simulink model "sim_sys2"  (R2013b)
settings: Solver=ode45  StartTime=0.0  StopTime=5000  RelTol=1e-3
undefined symbols (not defined in the file or in its folder): msdft_comb, resonator, sys_lib, twiddle_factors
libraries: xbsIndex_r4 x3996, casper_library_misc x310, xps_library x1
(part 1 of 46)
settings Model: Creator=root  LastModifiedBy=root

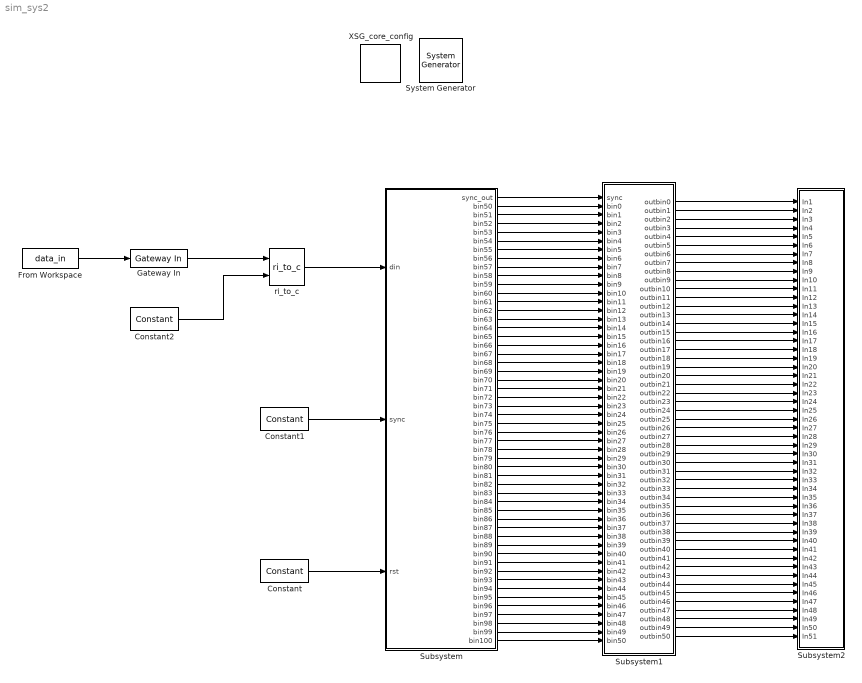
== system sim_sys2 ==
  " System Generator" : xbsIndex_r4/ System Generator  Tag=genX  xilinxfamily=Kintex7  part=xc7k325t  speed=-3  package=fbg676  synthesis_tool=XST  clock_wrapper=Clock Enables  directory=./netlist  proj_type=Project Navigator  Synth_file=XST Defaults  Impl_file=ISE Defaults  testbench=off  simulink_period=1  sysclk_period=10  dcm_input_clock_period=10  incr_netlist=off  trim_vbits=Everywhere in SubSystem  dbl_ovrd=According to Block Masks  core_generation=According to Block Masks  run_coregen=off  deprecated_control=off  eval_field=0  block_type=sysgen
  Constant : xbsIndex_r4/Constant  const=0  gui_display_data_type=Boolean  arith_type=Boolean  n_bits=16  bin_pt=14  preci_type=Single  exp_width=8  frac_width=24  explicit_period=on  period=1  equ=P=C  opselect=C  inp2=PCIN>>17  opr=+  inp1=P  carry=CIN  dbl_ovrd=off  block_type=constant
  Constant1 : xbsIndex_r4/Constant  const=1  gui_display_data_type=Boolean  arith_type=Boolean  n_bits=16  bin_pt=14  preci_type=Single  exp_width=8  frac_width=24  explicit_period=on  period=1  equ=P=C  opselect=C  inp2=PCIN>>17  opr=+  inp1=P  carry=CIN  dbl_ovrd=off  block_type=constant
  Constant2 : xbsIndex_r4/Constant  const=0  gui_display_data_type=Fixed-point  arith_type=Signed (2's comp)  n_bits=10  bin_pt=9  preci_type=Single  exp_width=8  frac_width=24  explicit_period=on  period=1  equ=P=C  opselect=C  inp2=PCIN>>17  opr=+  inp1=P  carry=CIN  dbl_ovrd=off  block_type=constant
  From Workspace : FromWorkspace  VariableName=data_in  SampleTime=0
  Gateway In : xbsIndex_r4/Gateway In  gui_display_data_type=Fixed-point  arith_type="Signed  (2's comp)"  n_bits=10  bin_pt=9  preci_type=Single  exp_width=8  frac_width=24  quantization="Round  (unbiased: +/- Inf)"  overflow=Saturate  period=1  dbl_ovrd=off  timing_constraint=None  locs_specified=off  LOCs={}  UseAsADC=off  ADCChannel='1'  inherit_from_input=off  hdl_port=on  block_type=gatewayin
  Subsystem : Subsystem  mask{input_bitsize=10, fft_len=10, bin_range=[50:1:100], twid_bitsize=15, res_out_size=40, out_bitsize=60, latency=0}
      mask prompts: input_bitsize "input bitsize"; fft_len "fft len (2^?)"; bin_range "bins"; res_out_size "resonator output"
      mask init:
      | config.source = str2func('msdft2_init');
      | config.toplevel = gcb;
      | xBlock(config, {input_bitsize, fft_len, bin_range,...
      |             twid_bitsize, res_out_size, ...
      |             out_bitsize, latency});
  Subsystem1 : Subsystem  mask{bin_len=51, bitwidth=40}
      mask prompts: bin_len "bin length"; bitwidth "bit width"
      mask init:
      | config.source = str2func('init_gate');
      | config.toplevel = gcb;
      | xBlock(config, {bin_len, bitwidth});
  Subsystem2 : Subsystem
  XSG_core_config : xps_library/XSG_core_config  Tag=xps:xsg  hw_sys=ROACH2:sx475t  clk_src=sys_clk  ROACH_clk_src=sys_clk  ROACH2_clk_src=sys_clk  MKDIG_clk_src=sys_clk  clk_rate=100  sample_period=1  synthesis_tool=XST
  ri_to_c : casper_library_misc/ri_to_c
  wires:
  Subsystem/52(bin100) -> Subsystem1/52(bin50)
  Subsystem/51(bin99) -> Subsystem1/51(bin49)
  Subsystem/50(bin98) -> Subsystem1/50(bin48)
  Subsystem/49(bin97) -> Subsystem1/49(bin47)
  Subsystem/48(bin96) -> Subsystem1/48(bin46)
  Subsystem/47(bin95) -> Subsystem1/47(bin45)
  Subsystem/45(bin93) -> Subsystem1/45(bin43)
  Subsystem/46(bin94) -> Subsystem1/46(bin44)
  Subsystem/44(bin92) -> Subsystem1/44(bin42)
  Subsystem/43(bin91) -> Subsystem1/43(bin41)
  Subsystem/42(bin90) -> Subsystem1/42(bin40)
  Subsystem/41(bin89) -> Subsystem1/41(bin39)
  Subsystem/40(bin88) -> Subsystem1/40(bin38)
  Subsystem/39(bin87) -> Subsystem1/39(bin37)
  Subsystem/38(bin86) -> Subsystem1/38(bin36)
  Subsystem/37(bin85) -> Subsystem1/37(bin35)
  Subsystem/36(bin84) -> Subsystem1/36(bin34)
  Subsystem/35(bin83) -> Subsystem1/35(bin33)
  Subsystem/34(bin82) -> Subsystem1/34(bin32)
  Subsystem/33(bin81) -> Subsystem1/33(bin31)
  Subsystem/32(bin80) -> Subsystem1/32(bin30)
  Subsystem/31(bin79) -> Subsystem1/31(bin29)
  Subsystem/30(bin78) -> Subsystem1/30(bin28)
  Subsystem/29(bin77) -> Subsystem1/29(bin27)
  Subsystem/28(bin76) -> Subsystem1/28(bin26)
  Subsystem/27(bin75) -> Subsystem1/27(bin25)
  Subsystem/26(bin74) -> Subsystem1/26(bin24)
  Subsystem/25(bin73) -> Subsystem1/25(bin23)
  Subsystem/24(bin72) -> Subsystem1/24(bin22)
  Subsystem/23(bin71) -> Subsystem1/23(bin21)
  Subsystem/22(bin70) -> Subsystem1/22(bin20)
  Subsystem/21(bin69) -> Subsystem1/21(bin19)
  Subsystem/20(bin68) -> Subsystem1/20(bin18)
  Subsystem/19(bin67) -> Subsystem1/19(bin17)
  Subsystem/18(bin66) -> Subsystem1/18(bin16)
  Subsystem/17(bin65) -> Subsystem1/17(bin15)
  Subsystem/16(bin64) -> Subsystem1/16(bin14)
  Subsystem/15(bin63) -> Subsystem1/15(bin13)
  Subsystem/14(bin62) -> Subsystem1/14(bin12)
  Subsystem/13(bin61) -> Subsystem1/13(bin11)
  Subsystem/12(bin60) -> Subsystem1/12(bin10)
  Subsystem/11(bin59) -> Subsystem1/11(bin9)
  Subsystem/10(bin58) -> Subsystem1/10(bin8)
  Subsystem/9(bin57) -> Subsystem1/9(bin7)
  Subsystem/8(bin56) -> Subsystem1/8(bin6)
  Subsystem/7(bin55) -> Subsystem1/7(bin5)
  Subsystem/6(bin54) -> Subsystem1/6(bin4)
  Subsystem/5(bin53) -> Subsystem1/5(bin3)
  Subsystem/4(bin52) -> Subsystem1/4(bin2)
  Subsystem/3(bin51) -> Subsystem1/3(bin1)
  Subsystem/2(bin50) -> Subsystem1/2(bin0)
  Subsystem/1(sync_out) -> Subsystem1/1(sync)
  Constant/1 -> Subsystem/3(rst)
  Constant1/1 -> Subsystem/2(sync)
  ri_to_c/1 -> Subsystem/1(din)
  Gateway In/1 -> ri_to_c/1
  From Workspace/1 -> Gateway In/1
  Constant2/1 -> ri_to_c/2
  Subsystem1/26(outbin25) -> Subsystem2/26(In26)
  Subsystem1/19(outbin18) -> Subsystem2/19(In19)
  Subsystem1/20(outbin19) -> Subsystem2/20(In20)
  Subsystem1/37(outbin36) -> Subsystem2/37(In37)
  Subsystem1/49(outbin48) -> Subsystem2/49(In49)
  Subsystem1/45(outbin44) -> Subsystem2/45(In45)
  Subsystem1/32(outbin31) -> Subsystem2/32(In32)
  Subsystem1/6(outbin5) -> Subsystem2/6(In6)
  Subsystem1/44(outbin43) -> Subsystem2/44(In44)
  Subsystem1/39(outbin38) -> Subsystem2/39(In39)
  Subsystem1/15(outbin14) -> Subsystem2/15(In15)
  Subsystem1/14(outbin13) -> Subsystem2/14(In14)
  Subsystem1/11(outbin10) -> Subsystem2/11(In11)
  Subsystem1/50(outbin49) -> Subsystem2/50(In50)
  Subsystem1/2(outbin1) -> Subsystem2/2(In2)
  Subsystem1/38(outbin37) -> Subsystem2/38(In38)
  Subsystem1/23(outbin22) -> Subsystem2/23(In23)
  Subsystem1/51(outbin50) -> Subsystem2/51(In51)
  Subsystem1/3(outbin2) -> Subsystem2/3(In3)
  Subsystem1/41(outbin40) -> Subsystem2/41(In41)
  Subsystem1/40(outbin39) -> Subsystem2/40(In40)
  Subsystem1/4(outbin3) -> Subsystem2/4(In4)
  Subsystem1/36(outbin35) -> Subsystem2/36(In36)
  Subsystem1/1(outbin0) -> Subsystem2/1(In1)
  Subsystem1/9(outbin8) -> Subsystem2/9(In9)
  Subsystem1/31(outbin30) -> Subsystem2/31(In31)
  Subsystem1/17(outbin16) -> Subsystem2/17(In17)
  Subsystem1/46(outbin45) -> Subsystem2/46(In46)
  Subsystem1/35(outbin34) -> Subsystem2/35(In35)
  Subsystem1/5(outbin4) -> Subsystem2/5(In5)
  Subsystem1/22(outbin21) -> Subsystem2/22(In22)
  Subsystem1/12(outbin11) -> Subsystem2/12(In12)
  Subsystem1/33(outbin32) -> Subsystem2/33(In33)
  Subsystem1/13(outbin12) -> Subsystem2/13(In13)
  Subsystem1/24(outbin23) -> Subsystem2/24(In24)
  Subsystem1/34(outbin33) -> Subsystem2/34(In34)
  Subsystem1/47(outbin46) -> Subsystem2/47(In47)
  Subsystem1/27(outbin26) -> Subsystem2/27(In27)
  Subsystem1/30(outbin29) -> Subsystem2/30(In30)
  Subsystem1/43(outbin42) -> Subsystem2/43(In43)
  Subsystem1/10(outbin9) -> Subsystem2/10(In10)
  Subsystem1/28(outbin27) -> Subsystem2/28(In28)
  Subsystem1/42(outbin41) -> Subsystem2/42(In42)
  Subsystem1/21(outbin20) -> Subsystem2/21(In21)
  Subsystem1/16(outbin15) -> Subsystem2/16(In16)
  Subsystem1/25(outbin24) -> Subsystem2/25(In25)
  Subsystem1/18(outbin17) -> Subsystem2/18(In18)
  Subsystem1/29(outbin28) -> Subsystem2/29(In29)
  Subsystem1/8(outbin7) -> Subsystem2/8(In8)
  Subsystem1/7(outbin6) -> Subsystem2/7(In7)
  Subsystem1/48(outbin47) -> Subsystem2/48(In48)

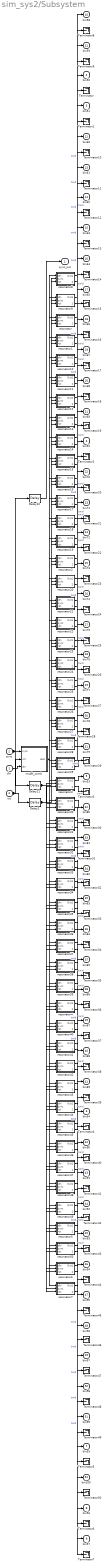
== system sim_sys2/Subsystem ==
  din : Inport
  sync : Inport  Port=2
  rst : Inport  Port=3
  Delay2 : xbsIndex_r4/Delay  rst=off  infoeditControl=Selection of Reset will increase slice count due to use of real FFs and instead of SRLs  en=off  latency=1  dbl_ovrd=off  reg_retiming=off  block_type=delay
  Delay21 : xbsIndex_r4/Delay  rst=off  infoeditControl=Selection of Reset will increase slice count due to use of real FFs and instead of SRLs  en=off  latency=1  dbl_ovrd=off  reg_retiming=off  block_type=delay
  Delay22 : xbsIndex_r4/Delay  rst=off  infoeditControl=Selection of Reset will increase slice count due to use of real FFs and instead of SRLs  en=off  latency=1036  dbl_ovrd=off  reg_retiming=off  block_type=delay
  Terminator{,1..50} (51 alike) : Terminator
  msdft_comb : Subsystem  AncestorBlock=sys_lib/msdft_comb  mask(msdft_comb){input_bitsize=10, fft_len=10, latency=0}
      mask prompts: fft_len "fft_len (2^?)"; latency "sub latency"
      mask init:
      | msdft_comb_init(gcb, ...
      |         'input_bitsize', input_bitsize, ...
      |         'fft_len', fft_len, ...
      |         'latency', latency);
      settings: AttributesFormatString=latency=0
  resonator : Subsystem  AncestorBlock=sys_lib/resonator  mask(msdft_res){fft_len=10, twid_bitsize=15, bin_number=50, input_bitsize=11, input_frac=9, res_bitsize=40, add_lat=0}
      mask prompts: fft_len "fft len(2^?)"; twid_bitsize "twid bitsize"; bin_number "bin number"; input_bitsize "input bitsize"; input_frac "input frac"; res_bitsize "out resonator size"
      mask init:
      | msdft_resonator_init(gcb, ...
      |                 'fft_len', fft_len, ...
      |                 'twid_bitsize', twid_bitsize, ...
      |                 'bin_number', bin_number, ...
      |                 'input_bitsize', input_bitsize, ...
      |                 'input_frac', input_frac, ...
      |                 'res_bitsize', res_bitsize, ...
      |                 'add_lat', add_lat);
      settings: AttributesFormatString=N=10, k=50
  resonator1 : Subsystem  AncestorBlock=sys_lib/resonator  mask(msdft_res){fft_len=10, twid_bitsize=15, bin_number=51, input_bitsize=11, input_frac=9, res_bitsize=40, add_lat=0}
      mask prompts: fft_len "fft len(2^?)"; twid_bitsize "twid bitsize"; bin_number "bin number"; input_bitsize "input bitsize"; input_frac "input frac"; res_bitsize "out resonator size"
      mask init: same as sim_sys2/Subsystem/resonator
      settings: AttributesFormatString=N=10, k=51
  resonator10 : Subsystem  AncestorBlock=sys_lib/resonator  mask(msdft_res){fft_len=10, twid_bitsize=15, bin_number=60, input_bitsize=11, input_frac=9, res_bitsize=40, add_lat=0}
      mask prompts: fft_len "fft len(2^?)"; twid_bitsize "twid bitsize"; bin_number "bin number"; input_bitsize "input bitsize"; input_frac "input frac"; res_bitsize "out resonator size"
      mask init: same as sim_sys2/Subsystem/resonator
      settings: AttributesFormatString=N=10, k=60
  resonator11 : Subsystem  AncestorBlock=sys_lib/resonator  mask(msdft_res){fft_len=10, twid_bitsize=15, bin_number=61, input_bitsize=11, input_frac=9, res_bitsize=40, add_lat=0}
      mask prompts: fft_len "fft len(2^?)"; twid_bitsize "twid bitsize"; bin_number "bin number"; input_bitsize "input bitsize"; input_frac "input frac"; res_bitsize "out resonator size"
      mask init: same as sim_sys2/Subsystem/resonator
      settings: AttributesFormatString=N=10, k=61
  resonator12 : Subsystem  AncestorBlock=sys_lib/resonator  mask(msdft_res){fft_len=10, twid_bitsize=15, bin_number=62, input_bitsize=11, input_frac=9, res_bitsize=40, add_lat=0}
      mask prompts: fft_len "fft len(2^?)"; twid_bitsize "twid bitsize"; bin_number "bin number"; input_bitsize "input bitsize"; input_frac "input frac"; res_bitsize "out resonator size"
      mask init: same as sim_sys2/Subsystem/resonator
      settings: AttributesFormatString=N=10, k=62
  resonator13 : Subsystem  AncestorBlock=sys_lib/resonator  mask(msdft_res){fft_len=10, twid_bitsize=15, bin_number=63, input_bitsize=11, input_frac=9, res_bitsize=40, add_lat=0}
      mask prompts: fft_len "fft len(2^?)"; twid_bitsize "twid bitsize"; bin_number "bin number"; input_bitsize "input bitsize"; input_frac "input frac"; res_bitsize "out resonator size"
      mask init: same as sim_sys2/Subsystem/resonator
      settings: AttributesFormatString=N=10, k=63
  resonator14 : Subsystem  AncestorBlock=sys_lib/resonator  mask(msdft_res){fft_len=10, twid_bitsize=15, bin_number=64, input_bitsize=11, input_frac=9, res_bitsize=40, add_lat=0}
      mask prompts: fft_len "fft len(2^?)"; twid_bitsize "twid bitsize"; bin_number "bin number"; input_bitsize "input bitsize"; input_frac "input frac"; res_bitsize "out resonator size"
      mask init: same as sim_sys2/Subsystem/resonator
      settings: AttributesFormatString=N=10, k=64
  resonator15 : Subsystem  AncestorBlock=sys_lib/resonator  mask(msdft_res){fft_len=10, twid_bitsize=15, bin_number=65, input_bitsize=11, input_frac=9, res_bitsize=40, add_lat=0}
      mask prompts: fft_len "fft len(2^?)"; twid_bitsize "twid bitsize"; bin_number "bin number"; input_bitsize "input bitsize"; input_frac "input frac"; res_bitsize "out resonator size"
      mask init: same as sim_sys2/Subsystem/resonator
      settings: AttributesFormatString=N=10, k=65
  resonator16 : Subsystem  AncestorBlock=sys_lib/resonator  mask(msdft_res){fft_len=10, twid_bitsize=15, bin_number=66, input_bitsize=11, input_frac=9, res_bitsize=40, add_lat=0}
      mask prompts: fft_len "fft len(2^?)"; twid_bitsize "twid bitsize"; bin_number "bin number"; input_bitsize "input bitsize"; input_frac "input frac"; res_bitsize "out resonator size"
      mask init: same as sim_sys2/Subsystem/resonator
      settings: AttributesFormatString=N=10, k=66
  resonator17 : Subsystem  AncestorBlock=sys_lib/resonator  mask(msdft_res){fft_len=10, twid_bitsize=15, bin_number=67, input_bitsize=11, input_frac=9, res_bitsize=40, add_lat=0}
      mask prompts: fft_len "fft len(2^?)"; twid_bitsize "twid bitsize"; bin_number "bin number"; input_bitsize "input bitsize"; input_frac "input frac"; res_bitsize "out resonator size"
      mask init: same as sim_sys2/Subsystem/resonator
      settings: AttributesFormatString=N=10, k=67
  resonator18 : Subsystem  AncestorBlock=sys_lib/resonator  mask(msdft_res){fft_len=10, twid_bitsize=15, bin_number=68, input_bitsize=11, input_frac=9, res_bitsize=40, add_lat=0}
      mask prompts: fft_len "fft len(2^?)"; twid_bitsize "twid bitsize"; bin_number "bin number"; input_bitsize "input bitsize"; input_frac "input frac"; res_bitsize "out resonator size"
      mask init: same as sim_sys2/Subsystem/resonator
      settings: AttributesFormatString=N=10, k=68
  resonator19 : Subsystem  AncestorBlock=sys_lib/resonator  mask(msdft_res){fft_len=10, twid_bitsize=15, bin_number=69, input_bitsize=11, input_frac=9, res_bitsize=40, add_lat=0}
      mask prompts: fft_len "fft len(2^?)"; twid_bitsize "twid bitsize"; bin_number "bin number"; input_bitsize "input bitsize"; input_frac "input frac"; res_bitsize "out resonator size"
      mask init: same as sim_sys2/Subsystem/resonator
      settings: AttributesFormatString=N=10, k=69
  resonator2 : Subsystem  AncestorBlock=sys_lib/resonator  mask(msdft_res){fft_len=10, twid_bitsize=15, bin_number=52, input_bitsize=11, input_frac=9, res_bitsize=40, add_lat=0}
      mask prompts: fft_len "fft len(2^?)"; twid_bitsize "twid bitsize"; bin_number "bin number"; input_bitsize "input bitsize"; input_frac "input frac"; res_bitsize "out resonator size"
      mask init: same as sim_sys2/Subsystem/resonator
      settings: AttributesFormatString=N=10, k=52
  resonator20 : Subsystem  AncestorBlock=sys_lib/resonator  mask(msdft_res){fft_len=10, twid_bitsize=15, bin_number=70, input_bitsize=11, input_frac=9, res_bitsize=40, add_lat=0}
      mask prompts: fft_len "fft len(2^?)"; twid_bitsize "twid bitsize"; bin_number "bin number"; input_bitsize "input bitsize"; input_frac "input frac"; res_bitsize "out resonator size"
      mask init: same as sim_sys2/Subsystem/resonator
      settings: AttributesFormatString=N=10, k=70
  resonator21 : Subsystem  AncestorBlock=sys_lib/resonator  mask(msdft_res){fft_len=10, twid_bitsize=15, bin_number=71, input_bitsize=11, input_frac=9, res_bitsize=40, add_lat=0}
      mask prompts: fft_len "fft len(2^?)"; twid_bitsize "twid bitsize"; bin_number "bin number"; input_bitsize "input bitsize"; input_frac "input frac"; res_bitsize "out resonator size"
      mask init: same as sim_sys2/Subsystem/resonator
      settings: AttributesFormatString=N=10, k=71
  resonator22 : Subsystem  AncestorBlock=sys_lib/resonator  mask(msdft_res){fft_len=10, twid_bitsize=15, bin_number=72, input_bitsize=11, input_frac=9, res_bitsize=40, add_lat=0}
      mask prompts: fft_len "fft len(2^?)"; twid_bitsize "twid bitsize"; bin_number "bin number"; input_bitsize "input bitsize"; input_frac "input frac"; res_bitsize "out resonator size"
      mask init: same as sim_sys2/Subsystem/resonator
      settings: AttributesFormatString=N=10, k=72
  resonator23 : Subsystem  AncestorBlock=sys_lib/resonator  mask(msdft_res){fft_len=10, twid_bitsize=15, bin_number=73, input_bitsize=11, input_frac=9, res_bitsize=40, add_lat=0}
      mask prompts: fft_len "fft len(2^?)"; twid_bitsize "twid bitsize"; bin_number "bin number"; input_bitsize "input bitsize"; input_frac "input frac"; res_bitsize "out resonator size"
      mask init: same as sim_sys2/Subsystem/resonator
      settings: AttributesFormatString=N=10, k=73
  resonator24 : Subsystem  AncestorBlock=sys_lib/resonator  mask(msdft_res){fft_len=10, twid_bitsize=15, bin_number=74, input_bitsize=11, input_frac=9, res_bitsize=40, add_lat=0}
      mask prompts: fft_len "fft len(2^?)"; twid_bitsize "twid bitsize"; bin_number "bin number"; input_bitsize "input bitsize"; input_frac "input frac"; res_bitsize "out resonator size"
      mask init: same as sim_sys2/Subsystem/resonator
      settings: AttributesFormatString=N=10, k=74
  resonator25 : Subsystem  AncestorBlock=sys_lib/resonator  mask(msdft_res){fft_len=10, twid_bitsize=15, bin_number=75, input_bitsize=11, input_frac=9, res_bitsize=40, add_lat=0}
      mask prompts: fft_len "fft len(2^?)"; twid_bitsize "twid bitsize"; bin_number "bin number"; input_bitsize "input bitsize"; input_frac "input frac"; res_bitsize "out resonator size"
      mask init: same as sim_sys2/Subsystem/resonator
      settings: AttributesFormatString=N=10, k=75
  resonator26 : Subsystem  AncestorBlock=sys_lib/resonator  mask(msdft_res){fft_len=10, twid_bitsize=15, bin_number=76, input_bitsize=11, input_frac=9, res_bitsize=40, add_lat=0}
      mask prompts: fft_len "fft len(2^?)"; twid_bitsize "twid bitsize"; bin_number "bin number"; input_bitsize "input bitsize"; input_frac "input frac"; res_bitsize "out resonator size"
      mask init: same as sim_sys2/Subsystem/resonator
      settings: AttributesFormatString=N=10, k=76
  resonator27 : Subsystem  AncestorBlock=sys_lib/resonator  mask(msdft_res){fft_len=10, twid_bitsize=15, bin_number=77, input_bitsize=11, input_frac=9, res_bitsize=40, add_lat=0}
      mask prompts: fft_len "fft len(2^?)"; twid_bitsize "twid bitsize"; bin_number "bin number"; input_bitsize "input bitsize"; input_frac "input frac"; res_bitsize "out resonator size"
      mask init: same as sim_sys2/Subsystem/resonator
      settings: AttributesFormatString=N=10, k=77
  resonator28 : Subsystem  AncestorBlock=sys_lib/resonator  mask(msdft_res){fft_len=10, twid_bitsize=15, bin_number=78, input_bitsize=11, input_frac=9, res_bitsize=40, add_lat=0}
      mask prompts: fft_len "fft len(2^?)"; twid_bitsize "twid bitsize"; bin_number "bin number"; input_bitsize "input bitsize"; input_frac "input frac"; res_bitsize "out resonator size"
      mask init: same as sim_sys2/Subsystem/resonator
      settings: AttributesFormatString=N=10, k=78
  resonator29 : Subsystem  AncestorBlock=sys_lib/resonator  mask(msdft_res){fft_len=10, twid_bitsize=15, bin_number=79, input_bitsize=11, input_frac=9, res_bitsize=40, add_lat=0}
      mask prompts: fft_len "fft len(2^?)"; twid_bitsize "twid bitsize"; bin_number "bin number"; input_bitsize "input bitsize"; input_frac "input frac"; res_bitsize "out resonator size"
      mask init: same as sim_sys2/Subsystem/resonator
      settings: AttributesFormatString=N=10, k=79
  resonator3 : Subsystem  AncestorBlock=sys_lib/resonator  mask(msdft_res){fft_len=10, twid_bitsize=15, bin_number=53, input_bitsize=11, input_frac=9, res_bitsize=40, add_lat=0}
      mask prompts: fft_len "fft len(2^?)"; twid_bitsize "twid bitsize"; bin_number "bin number"; input_bitsize "input bitsize"; input_frac "input frac"; res_bitsize "out resonator size"
      mask init: same as sim_sys2/Subsystem/resonator
      settings: AttributesFormatString=N=10, k=53
  resonator30 : Subsystem  AncestorBlock=sys_lib/resonator  mask(msdft_res){fft_len=10, twid_bitsize=15, bin_number=80, input_bitsize=11, input_frac=9, res_bitsize=40, add_lat=0}
      mask prompts: fft_len "fft len(2^?)"; twid_bitsize "twid bitsize"; bin_number "bin number"; input_bitsize "input bitsize"; input_frac "input frac"; res_bitsize "out resonator size"
      mask init: same as sim_sys2/Subsystem/resonator
      settings: AttributesFormatString=N=10, k=80
  resonator31 : Subsystem  AncestorBlock=sys_lib/resonator  mask(msdft_res){fft_len=10, twid_bitsize=15, bin_number=81, input_bitsize=11, input_frac=9, res_bitsize=40, add_lat=0}
      mask prompts: fft_len "fft len(2^?)"; twid_bitsize "twid bitsize"; bin_number "bin number"; input_bitsize "input bitsize"; input_frac "input frac"; res_bitsize "out resonator size"
      mask init: same as sim_sys2/Subsystem/resonator
      settings: AttributesFormatString=N=10, k=81
  resonator32 : Subsystem  AncestorBlock=sys_lib/resonator  mask(msdft_res){fft_len=10, twid_bitsize=15, bin_number=82, input_bitsize=11, input_frac=9, res_bitsize=40, add_lat=0}
      mask prompts: fft_len "fft len(2^?)"; twid_bitsize "twid bitsize"; bin_number "bin number"; input_bitsize "input bitsize"; input_frac "input frac"; res_bitsize "out resonator size"
      mask init: same as sim_sys2/Subsystem/resonator
      settings: AttributesFormatString=N=10, k=82
  resonator33 : Subsystem  AncestorBlock=sys_lib/resonator  mask(msdft_res){fft_len=10, twid_bitsize=15, bin_number=83, input_bitsize=11, input_frac=9, res_bitsize=40, add_lat=0}
      mask prompts: fft_len "fft len(2^?)"; twid_bitsize "twid bitsize"; bin_number "bin number"; input_bitsize "input bitsize"; input_frac "input frac"; res_bitsize "out resonator size"
      mask init: same as sim_sys2/Subsystem/resonator
      settings: AttributesFormatString=N=10, k=83
  resonator34 : Subsystem  AncestorBlock=sys_lib/resonator  mask(msdft_res){fft_len=10, twid_bitsize=15, bin_number=84, input_bitsize=11, input_frac=9, res_bitsize=40, add_lat=0}
      mask prompts: fft_len "fft len(2^?)"; twid_bitsize "twid bitsize"; bin_number "bin number"; input_bitsize "input bitsize"; input_frac "input frac"; res_bitsize "out resonator size"
      mask init: same as sim_sys2/Subsystem/resonator
      settings: AttributesFormatString=N=10, k=84
  resonator35 : Subsystem  AncestorBlock=sys_lib/resonator  mask(msdft_res){fft_len=10, twid_bitsize=15, bin_number=85, input_bitsize=11, input_frac=9, res_bitsize=40, add_lat=0}
      mask prompts: fft_len "fft len(2^?)"; twid_bitsize "twid bitsize"; bin_number "bin number"; input_bitsize "input bitsize"; input_frac "input frac"; res_bitsize "out resonator size"
      mask init: same as sim_sys2/Subsystem/resonator
      settings: AttributesFormatString=N=10, k=85
  resonator36 : Subsystem  AncestorBlock=sys_lib/resonator  mask(msdft_res){fft_len=10, twid_bitsize=15, bin_number=86, input_bitsize=11, input_frac=9, res_bitsize=40, add_lat=0}
      mask prompts: fft_len "fft len(2^?)"; twid_bitsize "twid bitsize"; bin_number "bin number"; input_bitsize "input bitsize"; input_frac "input frac"; res_bitsize "out resonator size"
      mask init: same as sim_sys2/Subsystem/resonator
      settings: AttributesFormatString=N=10, k=86
  resonator37 : Subsystem  AncestorBlock=sys_lib/resonator  mask(msdft_res){fft_len=10, twid_bitsize=15, bin_number=87, input_bitsize=11, input_frac=9, res_bitsize=40, add_lat=0}
      mask prompts: fft_len "fft len(2^?)"; twid_bitsize "twid bitsize"; bin_number "bin number"; input_bitsize "input bitsize"; input_frac "input frac"; res_bitsize "out resonator size"
      mask init: same as sim_sys2/Subsystem/resonator
      settings: AttributesFormatString=N=10, k=87
  resonator38 : Subsystem  AncestorBlock=sys_lib/resonator  mask(msdft_res){fft_len=10, twid_bitsize=15, bin_number=88, input_bitsize=11, input_frac=9, res_bitsize=40, add_lat=0}
      mask prompts: fft_len "fft len(2^?)"; twid_bitsize "twid bitsize"; bin_number "bin number"; input_bitsize "input bitsize"; input_frac "input frac"; res_bitsize "out resonator size"
      mask init: same as sim_sys2/Subsystem/resonator
      settings: AttributesFormatString=N=10, k=88
  resonator39 : Subsystem  AncestorBlock=sys_lib/resonator  mask(msdft_res){fft_len=10, twid_bitsize=15, bin_number=89, input_bitsize=11, input_frac=9, res_bitsize=40, add_lat=0}
      mask prompts: fft_len "fft len(2^?)"; twid_bitsize "twid bitsize"; bin_number "bin number"; input_bitsize "input bitsize"; input_frac "input frac"; res_bitsize "out resonator size"
      mask init: same as sim_sys2/Subsystem/resonator
      settings: AttributesFormatString=N=10, k=89
  resonator4 : Subsystem  AncestorBlock=sys_lib/resonator  mask(msdft_res){fft_len=10, twid_bitsize=15, bin_number=54, input_bitsize=11, input_frac=9, res_bitsize=40, add_lat=0}
      mask prompts: fft_len "fft len(2^?)"; twid_bitsize "twid bitsize"; bin_number "bin number"; input_bitsize "input bitsize"; input_frac "input frac"; res_bitsize "out resonator size"
      mask init: same as sim_sys2/Subsystem/resonator
      settings: AttributesFormatString=N=10, k=54
  resonator40 : Subsystem  AncestorBlock=sys_lib/resonator  mask(msdft_res){fft_len=10, twid_bitsize=15, bin_number=90, input_bitsize=11, input_frac=9, res_bitsize=40, add_lat=0}
      mask prompts: fft_len "fft len(2^?)"; twid_bitsize "twid bitsize"; bin_number "bin number"; input_bitsize "input bitsize"; input_frac "input frac"; res_bitsize "out resonator size"
      mask init: same as sim_sys2/Subsystem/resonator
      settings: AttributesFormatString=N=10, k=90
  resonator41 : Subsystem  AncestorBlock=sys_lib/resonator  mask(msdft_res){fft_len=10, twid_bitsize=15, bin_number=91, input_bitsize=11, input_frac=9, res_bitsize=40, add_lat=0}
      mask prompts: fft_len "fft len(2^?)"; twid_bitsize "twid bitsize"; bin_number "bin number"; input_bitsize "input bitsize"; input_frac "input frac"; res_bitsize "out resonator size"
      mask init: same as sim_sys2/Subsystem/resonator
      settings: AttributesFormatString=N=10, k=91
  resonator42 : Subsystem  AncestorBlock=sys_lib/resonator  mask(msdft_res){fft_len=10, twid_bitsize=15, bin_number=92, input_bitsize=11, input_frac=9, res_bitsize=40, add_lat=0}
      mask prompts: fft_len "fft len(2^?)"; twid_bitsize "twid bitsize"; bin_number "bin number"; input_bitsize "input bitsize"; input_frac "input frac"; res_bitsize "out resonator size"
      mask init: same as sim_sys2/Subsystem/resonator
      settings: AttributesFormatString=N=10, k=92
  resonator43 : Subsystem  AncestorBlock=sys_lib/resonator  mask(msdft_res){fft_len=10, twid_bitsize=15, bin_number=93, input_bitsize=11, input_frac=9, res_bitsize=40, add_lat=0}
      mask prompts: fft_len "fft len(2^?)"; twid_bitsize "twid bitsize"; bin_number "bin number"; input_bitsize "input bitsize"; input_frac "input frac"; res_bitsize "out resonator size"
      mask init: same as sim_sys2/Subsystem/resonator
      settings: AttributesFormatString=N=10, k=93
  resonator44 : Subsystem  AncestorBlock=sys_lib/resonator  mask(msdft_res){fft_len=10, twid_bitsize=15, bin_number=94, input_bitsize=11, input_frac=9, res_bitsize=40, add_lat=0}
      mask prompts: fft_len "fft len(2^?)"; twid_bitsize "twid bitsize"; bin_number "bin number"; input_bitsize "input bitsize"; input_frac "input frac"; res_bitsize "out resonator size"
      mask init: same as sim_sys2/Subsystem/resonator
      settings: AttributesFormatString=N=10, k=94
  resonator45 : Subsystem  AncestorBlock=sys_lib/resonator  mask(msdft_res){fft_len=10, twid_bitsize=15, bin_number=95, input_bitsize=11, input_frac=9, res_bitsize=40, add_lat=0}
      mask prompts: fft_len "fft len(2^?)"; twid_bitsize "twid bitsize"; bin_number "bin number"; input_bitsize "input bitsize"; input_frac "input frac"; res_bitsize "out resonator size"
      mask init: same as sim_sys2/Subsystem/resonator
      settings: AttributesFormatString=N=10, k=95
  resonator46 : Subsystem  AncestorBlock=sys_lib/resonator  mask(msdft_res){fft_len=10, twid_bitsize=15, bin_number=96, input_bitsize=11, input_frac=9, res_bitsize=40, add_lat=0}
      mask prompts: fft_len "fft len(2^?)"; twid_bitsize "twid bitsize"; bin_number "bin number"; input_bitsize "input bitsize"; input_frac "input frac"; res_bitsize "out resonator size"
      mask init: same as sim_sys2/Subsystem/resonator
      settings: AttributesFormatString=N=10, k=96
  resonator47 : Subsystem  AncestorBlock=sys_lib/resonator  mask(msdft_res){fft_len=10, twid_bitsize=15, bin_number=97, input_bitsize=11, input_frac=9, res_bitsize=40, add_lat=0}
      mask prompts: fft_len "fft len(2^?)"; twid_bitsize "twid bitsize"; bin_number "bin number"; input_bitsize "input bitsize"; input_frac "input frac"; res_bitsize "out resonator size"
      mask init: same as sim_sys2/Subsystem/resonator
      settings: AttributesFormatString=N=10, k=97
  resonator48 : Subsystem  AncestorBlock=sys_lib/resonator  mask(msdft_res){fft_len=10, twid_bitsize=15, bin_number=98, input_bitsize=11, input_frac=9, res_bitsize=40, add_lat=0}
      mask prompts: fft_len "fft len(2^?)"; twid_bitsize "twid bitsize"; bin_number "bin number"; input_bitsize "input bitsize"; input_frac "input frac"; res_bitsize "out resonator size"
      mask init: same as sim_sys2/Subsystem/resonator
      settings: AttributesFormatString=N=10, k=98
  resonator49 : Subsystem  AncestorBlock=sys_lib/resonator  mask(msdft_res){fft_len=10, twid_bitsize=15, bin_number=99, input_bitsize=11, input_frac=9, res_bitsize=40, add_lat=0}
      mask prompts: fft_len "fft len(2^?)"; twid_bitsize "twid bitsize"; bin_number "bin number"; input_bitsize "input bitsize"; input_frac "input frac"; res_bitsize "out resonator size"
      mask init: same as sim_sys2/Subsystem/resonator
      settings: AttributesFormatString=N=10, k=99
  resonator5 : Subsystem  AncestorBlock=sys_lib/resonator  mask(msdft_res){fft_len=10, twid_bitsize=15, bin_number=55, input_bitsize=11, input_frac=9, res_bitsize=40, add_lat=0}
      mask prompts: fft_len "fft len(2^?)"; twid_bitsize "twid bitsize"; bin_number "bin number"; input_bitsize "input bitsize"; input_frac "input frac"; res_bitsize "out resonator size"
      mask init: same as sim_sys2/Subsystem/resonator
      settings: AttributesFormatString=N=10, k=55
  resonator50 : Subsystem  AncestorBlock=sys_lib/resonator  mask(msdft_res){fft_len=10, twid_bitsize=15, bin_number=100, input_bitsize=11, input_frac=9, res_bitsize=40, add_lat=0}
      mask prompts: fft_len "fft len(2^?)"; twid_bitsize "twid bitsize"; bin_number "bin number"; input_bitsize "input bitsize"; input_frac "input frac"; res_bitsize "out resonator size"
      mask init: same as sim_sys2/Subsystem/resonator
      settings: AttributesFormatString=N=10, k=100
  resonator6 : Subsystem  AncestorBlock=sys_lib/resonator  mask(msdft_res){fft_len=10, twid_bitsize=15, bin_number=56, input_bitsize=11, input_frac=9, res_bitsize=40, add_lat=0}
      mask prompts: fft_len "fft len(2^?)"; twid_bitsize "twid bitsize"; bin_number "bin number"; input_bitsize "input bitsize"; input_frac "input frac"; res_bitsize "out resonator size"
      mask init: same as sim_sys2/Subsystem/resonator
      settings: AttributesFormatString=N=10, k=56
  resonator7 : Subsystem  AncestorBlock=sys_lib/resonator  mask(msdft_res){fft_len=10, twid_bitsize=15, bin_number=57, input_bitsize=11, input_frac=9, res_bitsize=40, add_lat=0}
      mask prompts: fft_len "fft len(2^?)"; twid_bitsize "twid bitsize"; bin_number "bin number"; input_bitsize "input bitsize"; input_frac "input frac"; res_bitsize "out resonator size"
      mask init: same as sim_sys2/Subsystem/resonator
      settings: AttributesFormatString=N=10, k=57
  resonator8 : Subsystem  AncestorBlock=sys_lib/resonator  mask(msdft_res){fft_len=10, twid_bitsize=15, bin_number=58, input_bitsize=11, input_frac=9, res_bitsize=40, add_lat=0}
      mask prompts: fft_len "fft len(2^?)"; twid_bitsize "twid bitsize"; bin_number "bin number"; input_bitsize "input bitsize"; input_frac "input frac"; res_bitsize "out resonator size"
      mask init: same as sim_sys2/Subsystem/resonator
      settings: AttributesFormatString=N=10, k=58
  resonator9 : Subsystem  AncestorBlock=sys_lib/resonator  mask(msdft_res){fft_len=10, twid_bitsize=15, bin_number=59, input_bitsize=11, input_frac=9, res_bitsize=40, add_lat=0}
      mask prompts: fft_len "fft len(2^?)"; twid_bitsize "twid bitsize"; bin_number "bin number"; input_bitsize "input bitsize"; input_frac "input frac"; res_bitsize "out resonator size"
      mask init: same as sim_sys2/Subsystem/resonator
      settings: AttributesFormatString=N=10, k=59
  sync_out : Outport
  bin50 : Outport  Port=2
  bin51 : Outport  Port=3
  bin52 : Outport  Port=4
  bin53 : Outport  Port=5
  bin54 : Outport  Port=6
  bin55 : Outport  Port=7
  bin56 : Outport  Port=8
  bin57 : Outport  Port=9
  bin58 : Outport  Port=10
  bin59 : Outport  Port=11
  bin60 : Outport  Port=12
  bin61 : Outport  Port=13
  bin62 : Outport  Port=14
  bin63 : Outport  Port=15
  bin64 : Outport  Port=16
  bin65 : Outport  Port=17
  bin66 : Outport  Port=18
  bin67 : Outport  Port=19
  bin68 : Outport  Port=20
  bin69 : Outport  Port=21
  bin70 : Outport  Port=22
  bin71 : Outport  Port=23
  bin72 : Outport  Port=24
  bin73 : Outport  Port=25
  bin74 : Outport  Port=26
  bin75 : Outport  Port=27
  bin76 : Outport  Port=28
  bin77 : Outport  Port=29
  bin78 : Outport  Port=30
  bin79 : Outport  Port=31
  bin80 : Outport  Port=32
  bin81 : Outport  Port=33
  bin82 : Outport  Port=34
  bin83 : Outport  Port=35
  bin84 : Outport  Port=36
  bin85 : Outport  Port=37
  bin86 : Outport  Port=38
  bin87 : Outport  Port=39
  bin88 : Outport  Port=40
  bin89 : Outport  Port=41
  bin90 : Outport  Port=42
  bin91 : Outport  Port=43
  bin92 : Outport  Port=44
  bin93 : Outport  Port=45
  bin94 : Outport  Port=46
  bin95 : Outport  Port=47
  bin96 : Outport  Port=48
  bin97 : Outport  Port=49
  bin98 : Outport  Port=50
  bin99 : Outport  Port=51
  bin100 : Outport  Port=52
  wires:
  sync/1 -> Delay22/1, Delay21/1, msdft_comb/1(sync)
  rst/1 -> Delay2/1, msdft_comb/2(rst)
  msdft_comb/1(dout) -> resonator50/1(din), resonator49/1(din), resonator48/1(din), resonator47/1(din), resonator46/1(din), resonator45/1(din), resonator44/1(din), resonator43/1(din), resonator42/1(din), resonator41/1(din), resonator40/1(din), resonator39/1(din), resonator38/1(din), resonator37/1(din), resonator36/1(din), resonator35/1(din), resonator34/1(din), resonator33/1(din), resonator32/1(din), resonator31/1(din), resonator30/1(din), resonator29/1(din), resonator28/1(din), resonator27/1(din), resonator26/1(din), resonator25/1(din), resonator24/1(din), resonator23/1(din), resonator22/1(din), resonator21/1(din), resonator20/1(din), resonator19/1(din), resonator18/1(din), resonator17/1(din), resonator16/1(din), resonator15/1(din), resonator14/1(din), resonator13/1(din), resonator12/1(din), resonator11/1(din), resonator10/1(din), resonator9/1(din), resonator8/1(din), resonator7/1(din), resonator6/1(din), resonator5/1(din), resonator4/1(din), resonator3/1(din), resonator2/1(din), resonator1/1(din), resonator/1(din)
  Delay21/1 -> resonator50/2(sync), resonator49/2(sync), resonator48/2(sync), resonator47/2(sync), resonator46/2(sync), resonator45/2(sync), resonator44/2(sync), resonator43/2(sync), resonator42/2(sync), resonator41/2(sync), resonator40/2(sync), resonator39/2(sync), resonator38/2(sync), resonator37/2(sync), resonator36/2(sync), resonator35/2(sync), resonator34/2(sync), resonator33/2(sync), resonator32/2(sync), resonator31/2(sync), resonator30/2(sync), resonator29/2(sync), resonator28/2(sync), resonator27/2(sync), resonator26/2(sync), resonator25/2(sync), resonator24/2(sync), resonator23/2(sync), resonator22/2(sync), resonator21/2(sync), resonator20/2(sync), resonator19/2(sync), resonator18/2(sync), resonator17/2(sync), resonator16/2(sync), resonator15/2(sync), resonator14/2(sync), resonator13/2(sync), resonator12/2(sync), resonator11/2(sync), resonator10/2(sync), resonator9/2(sync), resonator8/2(sync), resonator7/2(sync), resonator6/2(sync), resonator5/2(sync), resonator4/2(sync), resonator3/2(sync), resonator2/2(sync), resonator1/2(sync), resonator/2(sync)
  Delay2/1 -> resonator50/3(rst), resonator49/3(rst), resonator48/3(rst), resonator47/3(rst), resonator46/3(rst), resonator45/3(rst), resonator44/3(rst), resonator43/3(rst), resonator42/3(rst), resonator41/3(rst), resonator40/3(rst), resonator39/3(rst), resonator38/3(rst), resonator37/3(rst), resonator36/3(rst), resonator35/3(rst), resonator34/3(rst), resonator33/3(rst), resonator32/3(rst), resonator31/3(rst), resonator30/3(rst), resonator29/3(rst), resonator28/3(rst), resonator27/3(rst), resonator26/3(rst), resonator25/3(rst), resonator24/3(rst), resonator23/3(rst), resonator22/3(rst), resonator21/3(rst), resonator20/3(rst), resonator19/3(rst), resonator18/3(rst), resonator17/3(rst), resonator16/3(rst), resonator15/3(rst), resonator14/3(rst), resonator13/3(rst), resonator12/3(rst), resonator11/3(rst), resonator10/3(rst), resonator9/3(rst), resonator8/3(rst), resonator7/3(rst), resonator6/3(rst), resonator5/3(rst), resonator4/3(rst), resonator3/3(rst), resonator2/3(rst), resonator1/3(rst), resonator/3(rst)
  resonator50/2(twidd) -> Terminator50/1  "twid"
  resonator50/1(Out1) -> bin100/1
  resonator49/2(twidd) -> Terminator49/1  "twid"
  resonator49/1(Out1) -> bin99/1
  resonator48/2(twidd) -> Terminator48/1  "twid"
  resonator48/1(Out1) -> bin98/1
  resonator47/2(twidd) -> Terminator47/1  "twid"
  resonator47/1(Out1) -> bin97/1
  resonator46/2(twidd) -> Terminator46/1  "twid"
  resonator46/1(Out1) -> bin96/1
  resonator45/2(twidd) -> Terminator45/1  "twid"
  resonator45/1(Out1) -> bin95/1
  resonator44/2(twidd) -> Terminator44/1  "twid"
  resonator44/1(Out1) -> bin94/1
  resonator43/2(twidd) -> Terminator43/1  "twid"
  resonator43/1(Out1) -> bin93/1
  resonator42/2(twidd) -> Terminator42/1  "twid"
  resonator42/1(Out1) -> bin92/1
  resonator41/2(twidd) -> Terminator41/1  "twid"
  resonator41/1(Out1) -> bin91/1
  resonator40/2(twidd) -> Terminator40/1  "twid"
  resonator40/1(Out1) -> bin90/1
  resonator39/2(twidd) -> Terminator39/1  "twid"
  resonator39/1(Out1) -> bin89/1
  resonator38/2(twidd) -> Terminator38/1  "twid"
  resonator38/1(Out1) -> bin88/1
  resonator37/2(twidd) -> Terminator37/1  "twid"
  resonator37/1(Out1) -> bin87/1
  resonator36/2(twidd) -> Terminator36/1  "twid"
  resonator36/1(Out1) -> bin86/1
  resonator35/2(twidd) -> Terminator35/1  "twid"
  resonator35/1(Out1) -> bin85/1
  resonator34/2(twidd) -> Terminator34/1  "twid"
  resonator34/1(Out1) -> bin84/1
  resonator33/2(twidd) -> Terminator33/1  "twid"
  resonator33/1(Out1) -> bin83/1
  resonator32/2(twidd) -> Terminator32/1  "twid"
  resonator32/1(Out1) -> bin82/1
  resonator31/2(twidd) -> Terminator31/1  "twid"
  resonator31/1(Out1) -> bin81/1
  resonator30/2(twidd) -> Terminator30/1  "twid"
  resonator30/1(Out1) -> bin80/1
  resonator29/2(twidd) -> Terminator29/1  "twid"
  resonator29/1(Out1) -> bin79/1
  resonator28/2(twidd) -> Terminator28/1  "twid"
  resonator28/1(Out1) -> bin78/1
  resonator27/2(twidd) -> Terminator27/1  "twid"
  resonator27/1(Out1) -> bin77/1
  resonator26/2(twidd) -> Terminator26/1  "twid"
  resonator26/1(Out1) -> bin76/1
  resonator25/2(twidd) -> Terminator25/1  "twid"
  resonator25/1(Out1) -> bin75/1
  resonator24/2(twidd) -> Terminator24/1  "twid"
  resonator24/1(Out1) -> bin74/1
  resonator23/2(twidd) -> Terminator23/1  "twid"
  resonator23/1(Out1) -> bin73/1
  resonator22/2(twidd) -> Terminator22/1  "twid"
  resonator22/1(Out1) -> bin72/1
  resonator21/2(twidd) -> Terminator21/1  "twid"
  resonator21/1(Out1) -> bin71/1
  resonator20/2(twidd) -> Terminator20/1  "twid"
  resonator20/1(Out1) -> bin70/1
  resonator19/2(twidd) -> Terminator19/1  "twid"
  resonator19/1(Out1) -> bin69/1
  resonator18/2(twidd) -> Terminator18/1  "twid"
  resonator18/1(Out1) -> bin68/1
  resonator17/2(twidd) -> Terminator17/1  "twid"
  resonator17/1(Out1) -> bin67/1
  resonator16/2(twidd) -> Terminator16/1  "twid"
  resonator16/1(Out1) -> bin66/1
  resonator15/2(twidd) -> Terminator15/1  "twid"
  resonator15/1(Out1) -> bin65/1
  resonator14/2(twidd) -> Terminator14/1  "twid"
  resonator14/1(Out1) -> bin64/1
  resonator13/2(twidd) -> Terminator13/1  "twid"
  resonator13/1(Out1) -> bin63/1
  resonator12/2(twidd) -> Terminator12/1  "twid"
  resonator12/1(Out1) -> bin62/1
  resonator11/2(twidd) -> Terminator11/1  "twid"
  resonator11/1(Out1) -> bin61/1
  resonator10/2(twidd) -> Terminator10/1  "twid"
  resonator10/1(Out1) -> bin60/1
  resonator9/2(twidd) -> Terminator9/1  "twid"
  resonator9/1(Out1) -> bin59/1
  resonator8/2(twidd) -> Terminator8/1  "twid"
  resonator8/1(Out1) -> bin58/1
  resonator7/2(twidd) -> Terminator7/1  "twid"
  resonator7/1(Out1) -> bin57/1
  resonator6/2(twidd) -> Terminator6/1  "twid"
  resonator6/1(Out1) -> bin56/1
  resonator5/2(twidd) -> Terminator5/1  "twid"
  resonator5/1(Out1) -> bin55/1
  resonator4/2(twidd) -> Terminator4/1  "twid"
  resonator4/1(Out1) -> bin54/1
  resonator3/2(twidd) -> Terminator3/1  "twid"
  resonator3/1(Out1) -> bin53/1
  resonator2/2(twidd) -> Terminator2/1  "twid"
  resonator2/1(Out1) -> bin52/1
  resonator1/2(twidd) -> Terminator1/1  "twid"
  resonator1/1(Out1) -> bin51/1
  resonator/2(twidd) -> Terminator/1  "twid"
  resonator/1(Out1) -> bin50/1
  Delay22/1 -> sync_out/1
  din/1 -> msdft_comb/3(din)
